simulink model "task9a_v23b"  (R2023b)
settings: Solver=VariableStepAuto  StartTime=0.0  StopTime=3  RelTol=1e-5
libraries: robotmaniplib x2, robotcorelib x1
settings Model: Creator=laith  LastModifiedBy=Nico
settings RTWCC: GPUComputeCapability=5.0

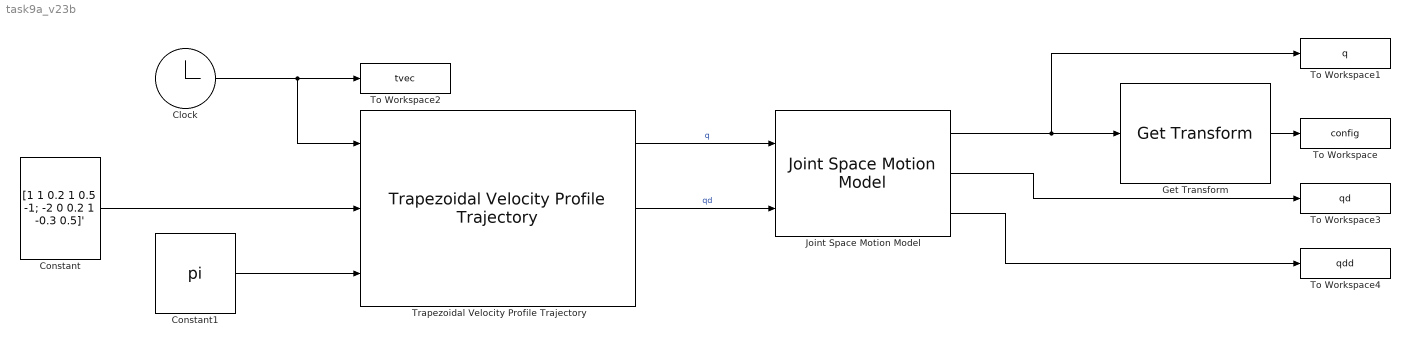
== system task9a_v23b ==
  " Joint Space Motion Model" : robotmaniplib/Joint Space Motion Model  RigidBodyTree=robotRBT  MotionType=PD Control  ProportionalGain=200  DerivativeGain=50  ErrorDynamicsSpecification=Damping Ratio / Natural Frequency  DampingRatio=1  NaturalFrequency=10  SettlingTime=0.59  Overshoot=0  ShowExternalForcePort=off  InitConfig="[1   1  0.2   1    0.5     -1]"  InitJointVel=0  SimulateUsing=Interpreted execution
  Clock : Clock
      settings: Decimation=100
  Constant : Constant  Value="[1   1  0.2   1    0.5     -1;  -2  0  0.2   1 -0.3    0.5]'"
  Constant1 : Constant  Value=pi
  Get Transform : robotmaniplib/Get Transform  RigidBodyTree=robotRBT  SourceBody=tool0  TargetBody=base_link  SimulateUsing=Interpreted execution
  To Workspace : ToWorkspace  VariableName=config  SampleTime=-1
  To Workspace1 : ToWorkspace  VariableName=q  SampleTime=-1
      settings: Save2DSignal=2-D array (concatenate along first dimension)
  To Workspace2 : ToWorkspace  VariableName=tvec  SampleTime=-1
  To Workspace3 : ToWorkspace  VariableName=qd  SampleTime=-1
      settings: Save2DSignal=2-D array (concatenate along first dimension)
  To Workspace4 : ToWorkspace  VariableName=qdd  SampleTime=-1
      settings: Save2DSignal=2-D array (concatenate along first dimension)
  Trapezoidal Velocity Profile Trajectory : robotcorelib/Trapezoidal Velocity Profile Trajectory  WaypointSource=External  Waypoints=[ 0, -0.5, -1; 0, 0.5, 1 ]  NumParams=1  Parameter1=Peak Velocity  Parameter2=Acceleration  ParameterSource=External  PeakVelocity=[ 2; 2 ]  Acceleration=[ 1; 2 ]  EndTime=[ 1; 1 ]  AccelTime=[ 1; 2 ]  SimulateUsing=Interpreted execution
  wires:
  Get Transform/1 -> To Workspace/1
  Constant1/1 -> Trapezoidal Velocity Profile Trajectory/3
  Constant/1 -> Trapezoidal Velocity Profile Trajectory/2
  Clock/1 -> Trapezoidal Velocity Profile Trajectory/1, To Workspace2/1
  " Joint Space Motion Model"/1 -> To Workspace1/1, Get Transform/1
  " Joint Space Motion Model"/2 -> To Workspace3/1
  " Joint Space Motion Model"/3 -> To Workspace4/1
  Trapezoidal Velocity Profile Trajectory/1 -> " Joint Space Motion Model"/1  "q"
  Trapezoidal Velocity Profile Trajectory/2 -> " Joint Space Motion Model"/2  "qd"
